simulink model "plots"  (R2024a)
settings: Solver=FixedStepAuto  StartTime=0.0  StopTime=120  FixedStep=0.01  RelTol=1e-3
values from neighbouring files (symbols this model uses):
  sc_size = 1    [Initiate_KUKA_inv.m]    (also in KUKA_Main.m)
settings Model: Creator=root  LastModifiedBy=Bmmog

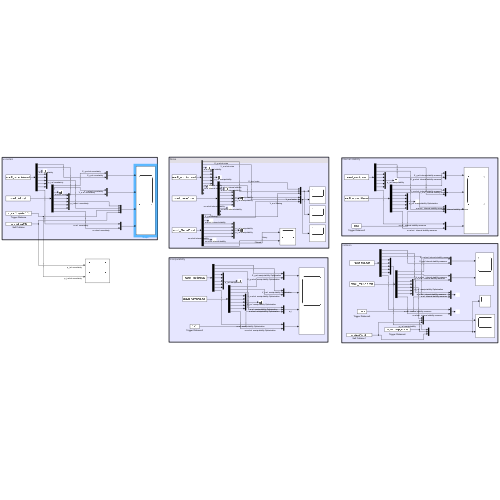
[thumbnail: Simulink's stored preview of the top-level diagram]
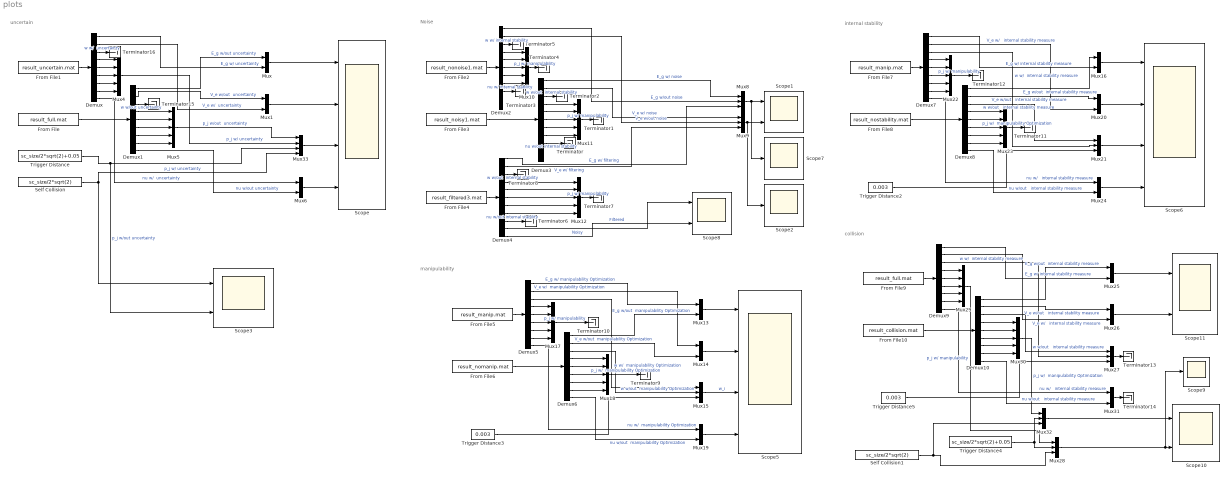
== system plots ==
  note: uncertain
  note: collision
  note: internal stability
  note: manipulability
  note: Noise
  Demux{,1,5..10} (8 alike) : Demux  Outputs=9
  Demux2 : Demux  Outputs=11
  Demux3 : Demux  Outputs=11
  Demux4 : Demux  Outputs=11
  From File : FromFile  FileName=result_full.mat  SampleTime=0
  From File1 : FromFile  FileName=result_uncertain.mat  SampleTime=0
  From File10 : FromFile  FileName=result_collision.mat  SampleTime=0
  From File2 : FromFile  FileName=result_nonoise1.mat  SampleTime=0
  From File3 : FromFile  FileName=result_noisy1.mat  SampleTime=0
  From File4 : FromFile  FileName=result_filtered3.mat  SampleTime=0
  From File5 : FromFile  FileName=result_manip.mat  SampleTime=0
  From File6 : FromFile  FileName=result_nomanip.mat  SampleTime=0
  From File7 : FromFile  FileName=result_manip.mat  SampleTime=0
  From File8 : FromFile  FileName=result_nostability.mat  SampleTime=0
  From File9 : FromFile  FileName=result_full.mat  SampleTime=0
  Mux{,1,6,13..14,16,19..20,24..26,31} (12 alike) : Mux  Inputs=2
  Mux{4..5,10..12,17..18,22..23,29..30} (11 alike) : Mux  Inputs=5
  Mux{8..9,15,21,27..28,32} (7 alike) : Mux  Inputs=3
  Mux33 : Mux
  Scope : Scope  NumInputPorts=4
  Scope{1,3,8,10..11} (5 alike) : Scope  NumInputPorts=2
  Scope2 : Scope
  Scope5 : Scope  NumInputPorts=4
  Scope6 : Scope  NumInputPorts=4
  Scope7 : Scope
  Scope9 : Scope
  Self Collision : Constant  Value=sc_size/2*sqrt(2)
  Self Collision1 : Constant  Value=sc_size/2*sqrt(2)
  Terminator{,1..16} (17 alike) : Terminator
  Trigger Distance : Constant  Value=sc_size/2*sqrt(2)+0.05
  Trigger Distance2 : Constant  Value=0.003
  Trigger Distance3 : Constant  Value=0.003
  Trigger Distance4 : Constant  Value=sc_size/2*sqrt(2)+0.05
  Trigger Distance5 : Constant  Value=0.003
  wires:
  Demux4/2 -> Mux9/3  "V_e w/ filtering"
  Demux4/9 -> Terminator6/1  "nu w/out internal stability"
  Demux4/7 -> Mux12/4
  Mux12/1 -> Terminator7/1  "p_j w/ manipulability"
  Demux4/1 -> Mux8/3  "E_g w/ filtering"
  From File4/1 -> Demux4/1
  Demux2/7 -> Mux10/4
  Demux2/3 -> Terminator5/1  "w w/ internal stability"
  Demux4/8 -> Mux12/5
  Demux3/6 -> Mux11/3
  Demux4/5 -> Mux12/2
  Mux11/1 -> Terminator1/1  "p_j w/ manipulability"
  Demux3/5 -> Mux11/2
  From File2/1 -> Demux2/1
  Demux2/8 -> Mux10/5
  Demux3/9 -> Terminator/1  "nu w/out internal stability"
  Demux3/1 -> Mux8/1  "E_g w/ noise"
  Demux3/7 -> Mux11/4
  Demux4/6 -> Mux12/3
  Mux9/1 -> Scope2/1, Scope1/2
  Demux2/5 -> Mux10/2
  Mux8/1 -> Scope7/1, Scope1/1
  Demux2/9 -> Terminator3/1  "nu w/ internal stability"
  Demux3/8 -> Mux11/5
  Demux2/2 -> Mux9/2  "V_e w/out noise"
  Demux3/2 -> Mux9/1  "V_e w/ noise"
  From File3/1 -> Demux3/1
  Mux10/1 -> Terminator4/1  "p_j w/ manipulability"
  Demux2/1 -> Mux8/2  "E_g w/out noise"
  Demux2/4 -> Mux10/1
  Demux3/3 -> Terminator2/1  "w w/out  internal stability"
  Demux4/4 -> Mux12/1
  Demux2/6 -> Mux10/3
  Demux4/3 -> Terminator8/1  "w w/out  internal stability"
  Demux3/4 -> Mux11/1
  From File6/1 -> Demux6/1
  Demux6/5 -> Mux18/2
  Demux6/9 -> Mux19/2  "nu w/out  manipulability Optimization"
  From File5/1 -> Demux5/1
  Demux6/8 -> Mux18/5
  Demux5/3 -> Mux15/1  "w w/  manipulability Optimization"
  Demux6/7 -> Mux18/4
  Trigger Distance3/1 -> Mux15/3
  Demux5/7 -> Mux17/4
  Demux6/4 -> Mux18/1
  Demux5/9 -> Mux19/1  "nu w/  manipulability Optimization"
  Demux5/6 -> Mux17/3
  Mux15/1 -> Scope5/3  "w_i"
  Demux6/6 -> Mux18/3
  Mux19/1 -> Scope5/4
  Demux5/5 -> Mux17/2
  Demux6/1 -> Mux13/2  "E_g w/out  manipulability Optimization"
  Demux6/3 -> Mux15/2  "w w/out  manipulability Optimization"
  Demux5/8 -> Mux17/5
  Demux6/2 -> Mux14/2  "V_e w/out  manipulability Optimization"
  Demux5/2 -> Mux14/1  "V_e w/  manipulability Optimization"
  Mux14/1 -> Scope5/2
  Demux5/1 -> Mux13/1  "E_g w/ manipulability Optimization"
  Demux5/4 -> Mux17/1
  Mux13/1 -> Scope5/1
  Mux18/1 -> Terminator9/1  "p_j w/  manipulability Optimization"
  Mux17/1 -> Terminator10/1  "p_j w/ manipulability"
  Demux8/1 -> Mux16/1  "E_g w/out  internal stability measure"
  Trigger Distance2/1 -> Mux21/3
  Demux7/8 -> Mux22/5
  Demux8/2 -> Mux20/1  "V_e w/out   internal stability measure"
  Demux8/8 -> Mux23/5
  From File7/1 -> Demux7/1
  Mux16/1 -> Scope6/1
  Demux7/9 -> Mux24/1  "nu w/   internal stability measure"
  Demux8/9 -> Mux24/2  "nu w/out   internal stability measure"
  Demux8/4 -> Mux23/1
  Mux20/1 -> Scope6/2
  Demux7/7 -> Mux22/4
  Demux7/6 -> Mux22/3
  From File8/1 -> Demux8/1
  Demux8/7 -> Mux23/4
  Demux8/6 -> Mux23/3
  Demux7/2 -> Mux20/2  "V_e w/   internal stability measure"
  Demux8/3 -> Mux21/1  "w w/out   internal stability measure"
  Mux21/1 -> Scope6/3
  Demux7/3 -> Mux21/2  "w w/  internal stability measure"
  Demux7/5 -> Mux22/2
  Demux7/4 -> Mux22/1
  Mux24/1 -> Scope6/4
  Demux8/5 -> Mux23/2
  Demux7/1 -> Mux16/2  "E_g w/ internal stability measure"
  Mux23/1 -> Terminator11/1  "p_j w/  manipulability Optimization"
  Mux22/1 -> Terminator12/1  "p_j w/ manipulability"
  Mux27/1 -> Terminator13/1
  From File10/1 -> Demux10/1
  From File9/1 -> Demux9/1
  Demux10/7 -> Mux30/4
  Demux10/6 -> Mux30/3
  Demux10/5 -> Mux30/2
  Self Collision1/1 -> Mux32/3, Mux28/3
  Demux9/5 -> Mux29/2
  Mux32/1 -> Scope10/1
  Demux9/1 -> Mux25/2  "E_g w/ internal stability measure"
  Demux9/4 -> Mux29/1
  Demux9/6 -> Mux29/3
  Trigger Distance4/1 -> Mux32/2, Mux28/2
  Mux28/1 -> Scope10/2, Scope9/1
  Demux10/9 -> Mux31/2  "nu w/out   internal stability measure"
  Mux31/1 -> Terminator14/1
  Demux9/7 -> Mux29/4
  Demux10/2 -> Mux26/1  "V_e w/out   internal stability measure"
  Mux26/1 -> Scope11/2
  Demux9/8 -> Mux29/5
  Mux25/1 -> Scope11/1
  Trigger Distance5/1 -> Mux27/3
  Demux10/8 -> Mux30/5
  Demux10/3 -> Mux27/1  "w w/out   internal stability measure"
  Demux9/3 -> Mux27/2  "w w/  internal stability measure"
  Demux10/4 -> Mux30/1
  Demux9/2 -> Mux26/2  "V_e w/   internal stability measure"
  Mux30/1 -> Mux32/1  "p_j w/  manipulability Optimization"
  Demux9/9 -> Mux31/1  "nu w/   internal stability measure"
  Mux29/1 -> Mux28/1  "p_j w/ manipulability"
  Demux10/1 -> Mux25/1  "E_g w/out  internal stability measure"
  Demux4/10 -> Scope8/1  "Noisy"
  Demux4/11 -> Scope8/2  "Filtered"
  Demux/3 -> Terminator16/1  "w w/  uncertainty"
  Mux6/1 -> Scope/4
  Demux/8 -> Mux4/5
  Mux5/1 -> Mux33/1  "p_j w/out  uncertainty"
  Demux1/9 -> Mux6/2  "nu w/out uncertainty"
  Demux/7 -> Mux4/4
  Demux/9 -> Mux6/1  "nu w/  uncertainty"
  Demux/1 -> Mux/2  "E_g w/ uncertainty"
  Demux/5 -> Mux4/2
  Demux1/8 -> Mux5/5
  Demux/2 -> Mux1/2  "V_e w/  uncertainty"
  Demux1/3 -> Terminator15/1  "w w/out uncertainty"
  Demux1/2 -> Mux1/1  "V_e w/out  uncertainty"
  Demux1/5 -> Mux5/2
  Demux1/1 -> Mux/1  "E_g w/out uncertainty"
  Demux1/7 -> Mux5/4
  Demux1/4 -> Mux5/1
  From File1/1 -> Demux/1
  Mux33/1 -> Scope/3
  Demux1/6 -> Mux5/3
  Mux/1 -> Scope/1
  Mux4/1 -> Mux33/2  "p_j w/ uncertainty"
  From File/1 -> Demux1/1
  Mux1/1 -> Scope/2
  Demux/6 -> Mux4/3
  Demux/4 -> Mux4/1
  Trigger Distance/1 -> Scope3/2, Mux33/3  "p_j w/out uncertainty"
  Self Collision/1 -> Mux33/4, Scope3/1  "p_j w/ uncertainty"
